simulink model "w3_warplab_agc"  (Simulink 7.7)
settings: Solver=ode45  StartTime=0.0  StopTime=1e4  RelTol=1e-3
PostLoadFcn:
  | w3_warplab_agc_init
InitFcn:
  | w3_warplab_agc_init
StartFcn:
  | w3_warplab_agc_init
values from neighbouring files (symbols this model uses):
  PHY_CONFIG_PKT_DET_CORR_THRESH = 90    [w3_warplab_agc_init.m]
  PHY_CONFIG_PKT_DET_ENERGY_THRESH = 14    [w3_warplab_agc_init.m]
  PHY_CONFIG_PKT_DET_MIN_DURR = 4    [w3_warplab_agc_init.m]
undefined symbols (not defined in the file or in its folder): gcbh, xlBlockLoadCallback, xlGetNormalizedPeriod
libraries: xbsIndex_r4 x1039, xbsEDKLib_r4 x1, simulink x1
(part 3 of 7)

== system w3_warplab_agc/Gain Calc A ==
  I : Inport
  Q : Inport  Port=2
  IQ Valid : Inport  Port=3
  RSSI : Inport  Port=4
  BB gain : Subsystem
  Capture & Convert : Subsystem
  IQ Mag : Subsystem
  RF Gain : Subsystem
  RSSI Avg : Subsystem
  Register{1..4} (4 alike) : xbsIndex_r4/Register  init=0  rst=off  en=off  dbl_ovrd=off  block_type=register
  G_RF : Outport
  G_BB : Outport  Port=2
  wires:
  RF Gain/1(G_RF) -> Register1/1, Capture & Convert/1(G_RF)
  Register1/1 -> Register2/1
  RSSI/1 -> RSSI Avg/1(RSSI)
  RSSI Avg/1(avg) -> Capture & Convert/2(RSSI)
  Capture & Convert/1(Rx Pwr (dBm)) -> RF Gain/1(Rx Pwr), BB gain/2(P_IN_RSSI)
  Register3/1 -> Register4/1
  BB gain/1(G_BB) -> Register3/1
  RF Gain/2(G_RF_dB) -> BB gain/1(G_RF_dB)
  IQ Mag/1(IQ_dBv) -> BB gain/3(IQ_dBv)
  I/1 -> IQ Mag/1(I)
  Q/1 -> IQ Mag/2(Q)
  IQ Valid/1 -> IQ Mag/3(Valid)
  Register2/1 -> G_RF/1
  Register4/1 -> G_BB/1

== system w3_warplab_agc/Gain Calc B ==
  I : Inport
  Q : Inport  Port=2
  IQ Valid : Inport  Port=3
  RSSI : Inport  Port=4
  BB gain : Subsystem
  Capture & Convert : Subsystem
  IQ Mag : Subsystem
  RF Gain : Subsystem
  RSSI Avg : Subsystem
  Register{1..4} (4 alike) : xbsIndex_r4/Register  init=0  rst=off  en=off  dbl_ovrd=off  block_type=register
  G_RF : Outport
  G_BB : Outport  Port=2
  wires:
  Register4/1 -> G_BB/1
  Register2/1 -> G_RF/1
  IQ Valid/1 -> IQ Mag/3(Valid)
  Q/1 -> IQ Mag/2(Q)
  I/1 -> IQ Mag/1(I)
  IQ Mag/1(IQ_dBv) -> BB gain/3(IQ_dBv)
  RF Gain/2(G_RF_dB) -> BB gain/1(G_RF_dB)
  BB gain/1(G_BB) -> Register3/1
  Register3/1 -> Register4/1
  Capture & Convert/1(Rx Pwr (dBm)) -> BB gain/2(P_IN_RSSI), RF Gain/1(Rx Pwr)
  RSSI Avg/1(avg) -> Capture & Convert/2(RSSI)
  RSSI/1 -> RSSI Avg/1(RSSI)
  Register1/1 -> Register2/1
  RF Gain/1(G_RF) -> Capture & Convert/1(G_RF), Register1/1

== system w3_warplab_agc/Gain Calc C ==
  I : Inport
  Q : Inport  Port=2
  IQ Valid : Inport  Port=3
  RSSI : Inport  Port=4
  BB gain : Subsystem
  Capture & Convert : Subsystem
  IQ Mag : Subsystem
  RF Gain : Subsystem
  RSSI Avg : Subsystem
  Register{1..4} (4 alike) : xbsIndex_r4/Register  init=0  rst=off  en=off  dbl_ovrd=off  block_type=register
  G_RF : Outport
  G_BB : Outport  Port=2
  wires:
  RF Gain/1(G_RF) -> Register1/1, Capture & Convert/1(G_RF)
  Register1/1 -> Register2/1
  RSSI/1 -> RSSI Avg/1(RSSI)
  RSSI Avg/1(avg) -> Capture & Convert/2(RSSI)
  Capture & Convert/1(Rx Pwr (dBm)) -> RF Gain/1(Rx Pwr), BB gain/2(P_IN_RSSI)
  Register3/1 -> Register4/1
  BB gain/1(G_BB) -> Register3/1
  RF Gain/2(G_RF_dB) -> BB gain/1(G_RF_dB)
  IQ Mag/1(IQ_dBv) -> BB gain/3(IQ_dBv)
  I/1 -> IQ Mag/1(I)
  Q/1 -> IQ Mag/2(Q)
  IQ Valid/1 -> IQ Mag/3(Valid)
  Register2/1 -> G_RF/1
  Register4/1 -> G_BB/1

== system w3_warplab_agc/Gain Calc D ==
  I : Inport
  Q : Inport  Port=2
  IQ Valid : Inport  Port=3
  RSSI : Inport  Port=4
  BB gain : Subsystem
  Capture & Convert : Subsystem
  IQ Mag : Subsystem
  RF Gain : Subsystem
  RSSI Avg : Subsystem
  Register{1..4} (4 alike) : xbsIndex_r4/Register  init=0  rst=off  en=off  dbl_ovrd=off  block_type=register
  G_RF : Outport
  G_BB : Outport  Port=2
  wires:
  Register4/1 -> G_BB/1
  Register2/1 -> G_RF/1
  IQ Valid/1 -> IQ Mag/3(Valid)
  Q/1 -> IQ Mag/2(Q)
  I/1 -> IQ Mag/1(I)
  IQ Mag/1(IQ_dBv) -> BB gain/3(IQ_dBv)
  RF Gain/2(G_RF_dB) -> BB gain/1(G_RF_dB)
  BB gain/1(G_BB) -> Register3/1
  Register3/1 -> Register4/1
  Capture & Convert/1(Rx Pwr (dBm)) -> BB gain/2(P_IN_RSSI), RF Gain/1(Rx Pwr)
  RSSI Avg/1(avg) -> Capture & Convert/2(RSSI)
  RSSI/1 -> RSSI Avg/1(RSSI)
  Register1/1 -> Register2/1
  RF Gain/1(G_RF) -> Capture & Convert/1(G_RF), Register1/1

== system w3_warplab_agc/IQ Outputs ==
  IQ Valid : Inport
  A I : Inport  Port=2
  A Q : Inport  Port=3
  B I : Inport  Port=4
  B Q : Inport  Port=5
  C I : Inport  Port=6
  C Q : Inport  Port=7
  D I : Inport  Port=8
  D Q : Inport  Port=9
  IQ_Valid_Out : xbsIndex_r4/Gateway Out  inherit_from_input=off  hdl_port=on  timing_constraint=None  locs_specified=off  LOCs={}  UseAsDAC=off  DACChannel='1'  block_type=gatewayout
  RFA_RX_I_OUT : xbsIndex_r4/Gateway Out  inherit_from_input=off  hdl_port=on  timing_constraint=None  locs_specified=off  LOCs={}  UseAsDAC=off  DACChannel='1'  block_type=gatewayout
  RFA_RX_Q_OUT : xbsIndex_r4/Gateway Out  inherit_from_input=off  hdl_port=on  timing_constraint=None  locs_specified=off  LOCs={}  UseAsDAC=off  DACChannel='1'  block_type=gatewayout
  RFB_RX_I_OUT : xbsIndex_r4/Gateway Out  inherit_from_input=off  hdl_port=on  timing_constraint=None  locs_specified=off  LOCs={}  UseAsDAC=off  DACChannel='1'  block_type=gatewayout
  RFB_RX_Q_OUT : xbsIndex_r4/Gateway Out  inherit_from_input=off  hdl_port=on  timing_constraint=None  locs_specified=off  LOCs={}  UseAsDAC=off  DACChannel='1'  block_type=gatewayout
  RFC_RX_I_OUT : xbsIndex_r4/Gateway Out  inherit_from_input=off  hdl_port=on  timing_constraint=None  locs_specified=off  LOCs={}  UseAsDAC=off  DACChannel='1'  block_type=gatewayout
  RFC_RX_Q_OUT : xbsIndex_r4/Gateway Out  inherit_from_input=off  hdl_port=on  timing_constraint=None  locs_specified=off  LOCs={}  UseAsDAC=off  DACChannel='1'  block_type=gatewayout
  RFD_RX_I_OUT : xbsIndex_r4/Gateway Out  inherit_from_input=off  hdl_port=on  timing_constraint=None  locs_specified=off  LOCs={}  UseAsDAC=off  DACChannel='1'  block_type=gatewayout
  RFD_RX_Q_OUT : xbsIndex_r4/Gateway Out  inherit_from_input=off  hdl_port=on  timing_constraint=None  locs_specified=off  LOCs={}  UseAsDAC=off  DACChannel='1'  block_type=gatewayout
  wires:
  A I/1 -> RFA_RX_I_OUT/1
  A Q/1 -> RFA_RX_Q_OUT/1
  IQ Valid/1 -> IQ_Valid_Out/1
  B I/1 -> RFB_RX_I_OUT/1
  B Q/1 -> RFB_RX_Q_OUT/1
  C I/1 -> RFC_RX_I_OUT/1
  C Q/1 -> RFC_RX_Q_OUT/1
  D I/1 -> RFD_RX_I_OUT/1
  D Q/1 -> RFD_RX_Q_OUT/1

== system w3_warplab_agc/RSSI Src ==
  Add : Sum
  Band-Limited White Noise : simulink/Sources/Band-Limited White Noise  SystemSampleTime=-1  Cov=200  Ts=1  seed=abs(ceil(1000*randn))
  Constant : Constant  Value=750
  Down Sample{,1..3} (4 alike) : xbsIndex_r4/Down Sample  sample_ratio=16  sample_phase="Last Value of Frame  (most efficient)"  en=off  latency=1  dbl_ovrd=off  block_type=dsamp
  RFA_RSSI : xbsIndex_r4/Gateway In  gui_display_data_type=Fixed-point  arith_type=Unsigned  n_bits=10  bin_pt=0  preci_type=Single  exp_width=8  frac_width=24  quantization="Round  (unbiased: +/- Inf)"  overflow=Saturate  period=1  dbl_ovrd=off  timing_constraint=None  locs_specified=off  LOCs={}  UseAsADC=off  ADCChannel='1'  inherit_from_input=off  hdl_port=on  block_type=gatewayin
  RFB_RSSI : xbsIndex_r4/Gateway In  gui_display_data_type=Fixed-point  arith_type=Unsigned  n_bits=10  bin_pt=0  preci_type=Single  exp_width=8  frac_width=24  quantization="Round  (unbiased: +/- Inf)"  overflow=Saturate  period=1  dbl_ovrd=off  timing_constraint=None  locs_specified=off  LOCs={}  UseAsADC=off  ADCChannel='1'  inherit_from_input=off  hdl_port=on  block_type=gatewayin
  RFC_RSSI : xbsIndex_r4/Gateway In  gui_display_data_type=Fixed-point  arith_type=Unsigned  n_bits=10  bin_pt=0  preci_type=Single  exp_width=8  frac_width=24  quantization="Round  (unbiased: +/- Inf)"  overflow=Saturate  period=1  dbl_ovrd=off  timing_constraint=None  locs_specified=off  LOCs={}  UseAsADC=off  ADCChannel='1'  inherit_from_input=off  hdl_port=on  block_type=gatewayin
  RFD_RSSI : xbsIndex_r4/Gateway In  gui_display_data_type=Fixed-point  arith_type=Unsigned  n_bits=10  bin_pt=0  preci_type=Single  exp_width=8  frac_width=24  quantization="Round  (unbiased: +/- Inf)"  overflow=Saturate  period=1  dbl_ovrd=off  timing_constraint=None  locs_specified=off  LOCs={}  UseAsADC=off  ADCChannel='1'  inherit_from_input=off  hdl_port=on  block_type=gatewayin
  Register{,1..3} (4 alike) : xbsIndex_r4/Register  init=0  rst=off  en=off  dbl_ovrd=off  block_type=register
  " RFA_RSSI" : Outport
  " RFB_RSSI" : Outport  Port=2
  " RFC_RSSI" : Outport  Port=3
  " RFD_RSSI" : Outport  Port=4
  wires:
  RFA_RSSI/1 -> Register/1
  Register/1 -> Down Sample/1
  Down Sample/1 -> " RFA_RSSI"/1
  Add/1 -> RFA_RSSI/1, RFB_RSSI/1, RFC_RSSI/1, RFD_RSSI/1
  Constant/1 -> Add/1
  Band-Limited White Noise/1 -> Add/2
  RFB_RSSI/1 -> Register1/1
  Register1/1 -> Down Sample1/1
  Down Sample1/1 -> " RFB_RSSI"/1
  RFC_RSSI/1 -> Register2/1
  RFD_RSSI/1 -> Register3/1
  Register2/1 -> Down Sample2/1
  Register3/1 -> Down Sample3/1
  Down Sample3/1 -> " RFD_RSSI"/1
  Down Sample2/1 -> " RFC_RSSI"/1

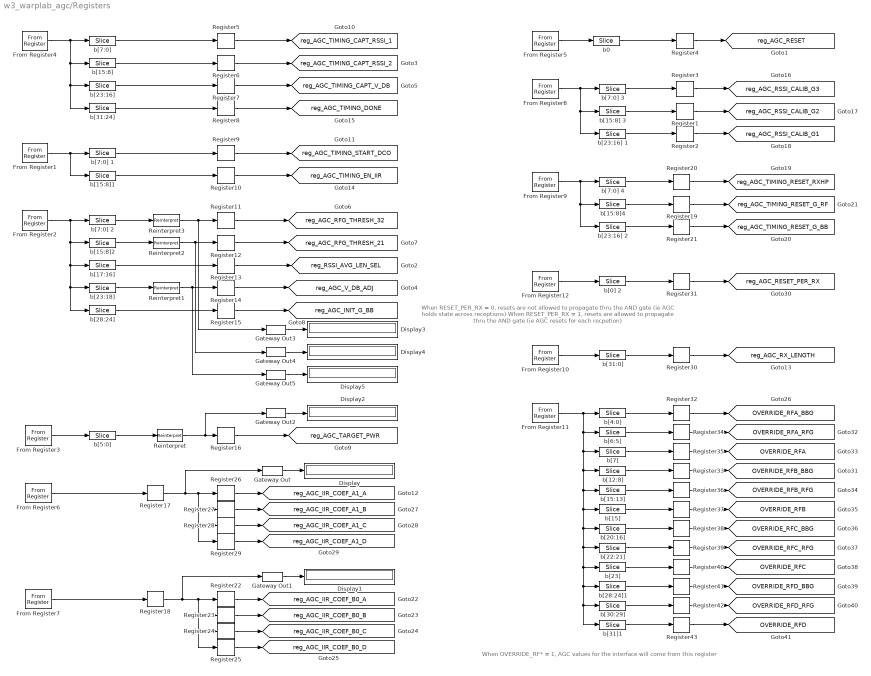
== system w3_warplab_agc/Registers ==
  note: When RESET_PER_RX = 0, resets are not allowed to propagate thru the AND gate (ie AGC holds state across receptions)
      | When RESET_PER_RX = 1, resets are allowed to propagate thru the AND gate (ie AGC resets for each recpetion)
  note: When OVERRIDE_RF* = 1, AGC values for the interface will come from this register
  Display{,1..5} (6 alike) : Display
  From Register1 : xbsIndex_r4/From Register  shared_memory_name='TIMING_DCO'  init=REG_AGC_Timing_DCO  period=1  ownership=Locally owned and initialized  gui_display_data_type=Fixed-point  arith_type=Unsigned  n_bits=32  bin_pt=0  preci_type=Single  dbl_ovrd=off  block_type=fromreg
      settings: AttributesFormatString=<< %<shared_memory_name> >>  infoedit="Register block that reads data to a shared memory register.  Delay of one sample period."
  From Register10 : xbsIndex_r4/From Register  shared_memory_name='RX_LENGTH'  init=REG_AGC_RX_LENGTH  period=1  ownership=Locally owned and initialized  gui_display_data_type=Fixed-point  arith_type=Unsigned  n_bits=32  bin_pt=0  preci_type=Single  dbl_ovrd=off  block_type=fromreg
      settings: AttributesFormatString=<< %<shared_memory_name> >>  infoedit="Register block that reads data to a shared memory register.  Delay of one sample period."
  From Register11 : xbsIndex_r4/From Register  shared_memory_name='AGC_OVERRIDE'  init=REG_ACG_OVERRIDE  period=1  ownership=Locally owned and initialized  gui_display_data_type=Fixed-point  arith_type=Unsigned  n_bits=32  bin_pt=0  preci_type=Single  dbl_ovrd=off  block_type=fromreg
      settings: AttributesFormatString=<< %<shared_memory_name> >>  infoedit="Register block that reads data to a shared memory register.  Delay of one sample period."
  From Register12 : xbsIndex_r4/From Register  shared_memory_name='RESET_MODE'  init=REG_AGC_RESET_MODE  period=1  ownership=Locally owned and initialized  gui_display_data_type=Fixed-point  arith_type=Unsigned  n_bits=32  bin_pt=0  preci_type=Single  dbl_ovrd=off  block_type=fromreg
      settings: AttributesFormatString=<< %<shared_memory_name> >>  infoedit="Register block that reads data to a shared memory register.  Delay of one sample period."
  From Register2 : xbsIndex_r4/From Register  shared_memory_name='CONFIG'  init=REG_AGC_Config  period=1  ownership=Locally owned and initialized  gui_display_data_type=Fixed-point  arith_type=Unsigned  n_bits=32  bin_pt=0  preci_type=Single  dbl_ovrd=off  block_type=fromreg
      settings: AttributesFormatString=<< %<shared_memory_name> >>  infoedit="Register block that reads data to a shared memory register.  Delay of one sample period."
  From Register3 : xbsIndex_r4/From Register  shared_memory_name='TARGET'  init=REG_AGC_Target  period=1  ownership=Locally owned and initialized  gui_display_data_type=Fixed-point  arith_type=Unsigned  n_bits=32  bin_pt=0  preci_type=Single  dbl_ovrd=off  block_type=fromreg
      settings: AttributesFormatString=<< %<shared_memory_name> >>  infoedit="Register block that reads data to a shared memory register.  Delay of one sample period."
  From Register4 : xbsIndex_r4/From Register  shared_memory_name='TIMING_AGC'  init=REG_AGC_Timing_AGC  period=1  ownership=Locally owned and initialized  gui_display_data_type=Fixed-point  arith_type=Unsigned  n_bits=32  bin_pt=0  preci_type=Single  dbl_ovrd=off  block_type=fromreg
      settings: AttributesFormatString=<< %<shared_memory_name> >>  infoedit="Register block that reads data to a shared memory register.  Delay of one sample period."
  From Register5 : xbsIndex_r4/From Register  shared_memory_name='RESET'  init=0  period=1  ownership=Locally owned and initialized  gui_display_data_type=Fixed-point  arith_type=Unsigned  n_bits=32  bin_pt=0  preci_type=Single  dbl_ovrd=off  block_type=fromreg
      settings: AttributesFormatString=<< %<shared_memory_name> >>  infoedit="Register block that reads data to a shared memory register.  Delay of one sample period."
  From Register6 : xbsIndex_r4/From Register  shared_memory_name='IIR_COEF_A1'  init=REG_AGC_IIR_Coef_A1  period=1  ownership=Locally owned and initialized  gui_display_data_type=Fixed-point  arith_type="Signed  (2's comp)"  n_bits=18  bin_pt=17  preci_type=Single  dbl_ovrd=off  block_type=fromreg
      settings: AttributesFormatString=<< %<shared_memory_name> >>  infoedit="Register block that reads data to a shared memory register.  Delay of one sample period."
  From Register7 : xbsIndex_r4/From Register  shared_memory_name='IIR_COEF_B0'  init=REG_AGC_IIR_Coef_B0  period=1  ownership=Locally owned and initialized  gui_display_data_type=Fixed-point  arith_type=Unsigned  n_bits=18  bin_pt=17  preci_type=Single  dbl_ovrd=off  block_type=fromreg
      settings: AttributesFormatString=<< %<shared_memory_name> >>  infoedit="Register block that reads data to a shared memory register.  Delay of one sample period."
  From Register8 : xbsIndex_r4/From Register  shared_memory_name='RSSI_PWR_CALIB'  init=REG_AGC_RSSI_RX_PWR_CALIB  period=1  ownership=Locally owned and initialized  gui_display_data_type=Fixed-point  arith_type=Unsigned  n_bits=32  bin_pt=0  preci_type=Single  dbl_ovrd=off  block_type=fromreg
      settings: AttributesFormatString=<< %<shared_memory_name> >>  infoedit="Register block that reads data to a shared memory register.  Delay of one sample period."
  From Register9 : xbsIndex_r4/From Register  shared_memory_name='TIMING_RESET'  init=REG_AGC_Timing_Reset  period=1  ownership=Locally owned and initialized  gui_display_data_type=Fixed-point  arith_type=Unsigned  n_bits=32  bin_pt=0  preci_type=Single  dbl_ovrd=off  block_type=fromreg
      settings: AttributesFormatString=<< %<shared_memory_name> >>  infoedit="Register block that reads data to a shared memory register.  Delay of one sample period."
  Gateway Out{,1..5} (6 alike) : xbsIndex_r4/Gateway Out  inherit_from_input=off  hdl_port=off  timing_constraint=None  locs_specified=off  LOCs={}  UseAsDAC=off  DACChannel='1'  block_type=gatewayout
  Register{1..43} (43 alike) : xbsIndex_r4/Register  init=0  rst=off  en=off  dbl_ovrd=off  block_type=register
  Reinterpret{,1..3} (4 alike) : xbsIndex_r4/Reinterpret  force_arith_type=on  arith_type="Signed  (2's comp)"  force_bin_pt=off  bin_pt=0  block_type=reinterpret
  b0 : xbsIndex_r4/Slice  nbits=1  boolean_output=on  mode=Lower Bit Location + Width  bit1=0  base1=MSB of Input  bit0=0  base0=LSB of Input  dbl_ovrd=off  block_type=slice
      settings: block_version=VER_STRING_GOES_HERE
  b[0] 2 : xbsIndex_r4/Slice  nbits=1  boolean_output=off  mode=Lower Bit Location + Width  bit1=0  base1=MSB of Input  bit0=0  base0=LSB of Input  dbl_ovrd=off  block_type=slice
      settings: block_version=VER_STRING_GOES_HERE
  b[12:8] : xbsIndex_r4/Slice  nbits=5  boolean_output=off  mode=Lower Bit Location + Width  bit1=0  base1=MSB of Input  bit0=8  base0=LSB of Input  dbl_ovrd=off  block_type=slice
      settings: block_version=VER_STRING_GOES_HERE
  b[15:13] : xbsIndex_r4/Slice  nbits=2  boolean_output=off  mode=Lower Bit Location + Width  bit1=0  base1=MSB of Input  bit0=13  base0=LSB of Input  dbl_ovrd=off  block_type=slice
      settings: block_version=VER_STRING_GOES_HERE
  b[15:8]{,1..2,4} (4 alike) : xbsIndex_r4/Slice  nbits=8  boolean_output=off  mode=Lower Bit Location + Width  bit1=0  base1=MSB of Input  bit0=8  base0=LSB of Input  dbl_ovrd=off  block_type=slice
      settings: block_version=VER_STRING_GOES_HERE
  b[15:8] 3 : xbsIndex_r4/Slice  nbits=8  boolean_output=off  mode=Lower Bit Location + Width  bit1=0  base1=MSB of Input  bit0=8  base0=LSB of Input  dbl_ovrd=off  block_type=slice
      settings: block_version=VER_STRING_GOES_HERE
  b[15] : xbsIndex_r4/Slice  nbits=1  boolean_output=off  mode=Lower Bit Location + Width  bit1=0  base1=MSB of Input  bit0=15  base0=LSB of Input  dbl_ovrd=off  block_type=slice
      settings: block_version=VER_STRING_GOES_HERE
  b[17:16] : xbsIndex_r4/Slice  nbits=2  boolean_output=off  mode=Lower Bit Location + Width  bit1=0  base1=MSB of Input  bit0=16  base0=LSB of Input  dbl_ovrd=off  block_type=slice
      settings: block_version=VER_STRING_GOES_HERE
  b[20:16] : xbsIndex_r4/Slice  nbits=5  boolean_output=off  mode=Lower Bit Location + Width  bit1=0  base1=MSB of Input  bit0=16  base0=LSB of Input  dbl_ovrd=off  block_type=slice
      settings: block_version=VER_STRING_GOES_HERE
  b[22:21] : xbsIndex_r4/Slice  nbits=2  boolean_output=off  mode=Lower Bit Location + Width  bit1=0  base1=MSB of Input  bit0=21  base0=LSB of Input  dbl_ovrd=off  block_type=slice
      settings: block_version=VER_STRING_GOES_HERE
  b[23:16] : xbsIndex_r4/Slice  nbits=8  boolean_output=off  mode=Lower Bit Location + Width  bit1=0  base1=MSB of Input  bit0=16  base0=LSB of Input  dbl_ovrd=off  block_type=slice
      settings: block_version=VER_STRING_GOES_HERE
  b[23:16] 1 : xbsIndex_r4/Slice  nbits=8  boolean_output=off  mode=Lower Bit Location + Width  bit1=0  base1=MSB of Input  bit0=16  base0=LSB of Input  dbl_ovrd=off  block_type=slice
      settings: block_version=VER_STRING_GOES_HERE
  b[23:16] 2 : xbsIndex_r4/Slice  nbits=8  boolean_output=off  mode=Lower Bit Location + Width  bit1=0  base1=MSB of Input  bit0=16  base0=LSB of Input  dbl_ovrd=off  block_type=slice
      settings: block_version=VER_STRING_GOES_HERE
  b[23:18] : xbsIndex_r4/Slice  nbits=6  boolean_output=off  mode=Lower Bit Location + Width  bit1=0  base1=MSB of Input  bit0=18  base0=LSB of Input  dbl_ovrd=off  block_type=slice
      settings: block_version=VER_STRING_GOES_HERE
  b[23] : xbsIndex_r4/Slice  nbits=1  boolean_output=off  mode=Lower Bit Location + Width  bit1=0  base1=MSB of Input  bit0=23  base0=LSB of Input  dbl_ovrd=off  block_type=slice
      settings: block_version=VER_STRING_GOES_HERE
  b[28:24] : xbsIndex_r4/Slice  nbits=5  boolean_output=off  mode=Lower Bit Location + Width  bit1=0  base1=MSB of Input  bit0=24  base0=LSB of Input  dbl_ovrd=off  block_type=slice
      settings: block_version=VER_STRING_GOES_HERE
  b[28:24]1 : xbsIndex_r4/Slice  nbits=5  boolean_output=off  mode=Lower Bit Location + Width  bit1=0  base1=MSB of Input  bit0=24  base0=LSB of Input  dbl_ovrd=off  block_type=slice
      settings: block_version=VER_STRING_GOES_HERE
  b[30:29] : xbsIndex_r4/Slice  nbits=2  boolean_output=off  mode=Lower Bit Location + Width  bit1=0  base1=MSB of Input  bit0=29  base0=LSB of Input  dbl_ovrd=off  block_type=slice
      settings: block_version=VER_STRING_GOES_HERE
  b[31:0] : xbsIndex_r4/Slice  nbits=32  boolean_output=off  mode=Lower Bit Location + Width  bit1=0  base1=MSB of Input  bit0=0  base0=LSB of Input  dbl_ovrd=off  block_type=slice
      settings: block_version=VER_STRING_GOES_HERE
  b[31:24] : xbsIndex_r4/Slice  nbits=8  boolean_output=off  mode=Lower Bit Location + Width  bit1=0  base1=MSB of Input  bit0=24  base0=LSB of Input  dbl_ovrd=off  block_type=slice
      settings: block_version=VER_STRING_GOES_HERE
  b[31]1 : xbsIndex_r4/Slice  nbits=1  boolean_output=off  mode=Lower Bit Location + Width  bit1=0  base1=MSB of Input  bit0=31  base0=LSB of Input  dbl_ovrd=off  block_type=slice
      settings: block_version=VER_STRING_GOES_HERE
  b[4:0] : xbsIndex_r4/Slice  nbits=5  boolean_output=off  mode=Lower Bit Location + Width  bit1=0  base1=MSB of Input  bit0=0  base0=LSB of Input  dbl_ovrd=off  block_type=slice
      settings: block_version=VER_STRING_GOES_HERE
  b[5:0] : xbsIndex_r4/Slice  nbits=6  boolean_output=off  mode=Lower Bit Location + Width  bit1=0  base1=MSB of Input  bit0=0  base0=LSB of Input  dbl_ovrd=off  block_type=slice
      settings: block_version=VER_STRING_GOES_HERE
  b[6:5] : xbsIndex_r4/Slice  nbits=2  boolean_output=off  mode=Lower Bit Location + Width  bit1=0  base1=MSB of Input  bit0=5  base0=LSB of Input  dbl_ovrd=off  block_type=slice
      settings: block_version=VER_STRING_GOES_HERE
  b[7:0] {,1..4} (5 alike) : xbsIndex_r4/Slice  nbits=8  boolean_output=off  mode=Lower Bit Location + Width  bit1=0  base1=MSB of Input  bit0=0  base0=LSB of Input  dbl_ovrd=off  block_type=slice
      settings: block_version=VER_STRING_GOES_HERE
  b[7] : xbsIndex_r4/Slice  nbits=1  boolean_output=off  mode=Lower Bit Location + Width  bit1=0  base1=MSB of Input  bit0=7  base0=LSB of Input  dbl_ovrd=off  block_type=slice
      settings: block_version=VER_STRING_GOES_HERE
  tag scope: OVERRIDE_RFA=global, OVERRIDE_RFA_BBG=global, OVERRIDE_RFA_RFG=global, OVERRIDE_RFB=global, OVERRIDE_RFB_BBG=global, OVERRIDE_RFB_RFG=global, OVERRIDE_RFC=global, OVERRIDE_RFC_BBG=global, OVERRIDE_RFC_RFG=global, OVERRIDE_RFD=global, OVERRIDE_RFD_BBG=global, OVERRIDE_RFD_RFG=global, reg_AGC_IIR_COEF_A1_A=global, reg_AGC_IIR_COEF_A1_B=global, reg_AGC_IIR_COEF_A1_C=global, reg_AGC_IIR_COEF_A1_D=global, reg_AGC_IIR_COEF_B0_A=global, reg_AGC_IIR_COEF_B0_B=global, reg_AGC_IIR_COEF_B0_C=global, reg_AGC_IIR_COEF_B0_D=global, reg_AGC_INIT_G_BB=global, reg_AGC_RESET=global, reg_AGC_RESET_PER_RX=global, reg_AGC_RFG_THRESH_21=global, reg_AGC_RFG_THRESH_32=global, reg_AGC_RSSI_CALIB_G1=global, reg_AGC_RSSI_CALIB_G2=global, reg_AGC_RSSI_CALIB_G3=global, reg_AGC_RX_LENGTH=global, reg_AGC_TARGET_PWR=global, reg_AGC_TIMING_CAPT_RSSI_1=global, reg_AGC_TIMING_CAPT_RSSI_2=global, reg_AGC_TIMING_CAPT_V_DB=global, reg_AGC_TIMING_DONE=global, reg_AGC_TIMING_EN_IIR=global, reg_AGC_TIMING_RESET_G_BB=global, reg_AGC_TIMING_RESET_G_RF=global, reg_AGC_TIMING_RESET_RXHP=global, reg_AGC_TIMING_START_DCO=global, reg_AGC_V_DB_ADJ=global, reg_RSSI_AVG_LEN_SEL=global
  wires:
  From Register4/1 -> "b[7:0] "/1, b[15:8]/1, b[23:16]/1, b[31:24]/1
  "b[7:0] "/1 -> Register5/1
  b[15:8]/1 -> Register6/1
  b[23:16]/1 -> Register7/1
  From Register1/1 -> b[7:0] 1/1, b[15:8]1/1
  b[7:0] 1/1 -> Register9/1
  b[15:8]1/1 -> Register10/1
  From Register2/1 -> b[15:8]2/1, b[17:16]/1, b[23:18]/1, b[28:24]/1, b[7:0] 2/1
  b[7:0] 2/1 -> Reinterpret3/1
  b[15:8]2/1 -> Reinterpret2/1
  b[17:16]/1 -> Register13/1
  b[23:18]/1 -> Reinterpret1/1
  b[28:24]/1 -> Register15/1
  From Register3/1 -> b[5:0]/1
  b[5:0]/1 -> Reinterpret/1
  Reinterpret/1 -> Gateway Out2/1, Register16/1
  Reinterpret1/1 -> Gateway Out5/1, Register14/1
  Reinterpret2/1 -> Gateway Out4/1, Register12/1
  Reinterpret3/1 -> Gateway Out3/1, Register11/1
  From Register5/1 -> b0/1
  b0/1 -> Register4/1
  From Register6/1 -> Register17/1
  From Register7/1 -> Register18/1
  Gateway Out/1 -> Display/1
  Gateway Out1/1 -> Display1/1
  Gateway Out2/1 -> Display2/1
  Gateway Out3/1 -> Display3/1
  Gateway Out4/1 -> Display4/1
  Gateway Out5/1 -> Display5/1
  b[31:24]/1 -> Register8/1
  From Register8/1 -> b[15:8] 3/1, b[23:16] 1/1, b[7:0] 3/1
  b[7:0] 3/1 -> Register3/1
  b[15:8] 3/1 -> Register1/1
  b[23:16] 1/1 -> Register2/1
  Register3/1 -> [reg_AGC_RSSI_CALIB_G3]
  Register1/1 -> [reg_AGC_RSSI_CALIB_G2]
  Register2/1 -> [reg_AGC_RSSI_CALIB_G1]
  Register4/1 -> [reg_AGC_RESET]
  Register5/1 -> [reg_AGC_TIMING_CAPT_RSSI_1]
  Register6/1 -> [reg_AGC_TIMING_CAPT_RSSI_2]
  Register7/1 -> [reg_AGC_TIMING_CAPT_V_DB]
  Register8/1 -> [reg_AGC_TIMING_DONE]
  Register9/1 -> [reg_AGC_TIMING_START_DCO]
  Register10/1 -> [reg_AGC_TIMING_EN_IIR]
  Register11/1 -> [reg_AGC_RFG_THRESH_32]
  Register12/1 -> [reg_AGC_RFG_THRESH_21]
  Register13/1 -> [reg_RSSI_AVG_LEN_SEL]
  Register14/1 -> [reg_AGC_V_DB_ADJ]
  Register15/1 -> [reg_AGC_INIT_G_BB]
  Register16/1 -> [reg_AGC_TARGET_PWR]
  Register17/1 -> Gateway Out/1, Register28/1, Register29/1, Register27/1, Register26/1
  Register18/1 -> Gateway Out1/1, Register24/1, Register25/1, Register23/1, Register22/1
  From Register9/1 -> b[7:0] 4/1, b[15:8]4/1, b[23:16] 2/1
  b[7:0] 4/1 -> Register20/1
  b[15:8]4/1 -> Register19/1
  Register20/1 -> [reg_AGC_TIMING_RESET_RXHP]
  Register19/1 -> [reg_AGC_TIMING_RESET_G_RF]
  b[23:16] 2/1 -> Register21/1
  Register21/1 -> [reg_AGC_TIMING_RESET_G_BB]
  Register22/1 -> [reg_AGC_IIR_COEF_B0_A]
  Register23/1 -> [reg_AGC_IIR_COEF_B0_B]
  Register24/1 -> [reg_AGC_IIR_COEF_B0_C]
  Register25/1 -> [reg_AGC_IIR_COEF_B0_D]
  Register26/1 -> [reg_AGC_IIR_COEF_A1_A]
  Register27/1 -> [reg_AGC_IIR_COEF_A1_B]
  Register28/1 -> [reg_AGC_IIR_COEF_A1_C]
  Register29/1 -> [reg_AGC_IIR_COEF_A1_D]
  From Register10/1 -> b[31:0]/1
  b[31:0]/1 -> Register30/1
  b[0] 2/1 -> Register31/1
  Register30/1 -> [reg_AGC_RX_LENGTH]
  Register31/1 -> [reg_AGC_RESET_PER_RX]
  From Register11/1 -> b[4:0]/1, b[6:5]/1, b[7]/1, b[12:8]/1, b[15:13]/1, b[15]/1, b[20:16]/1, b[22:21]/1, b[23]/1, b[28:24]1/1, b[30:29]/1, b[31]1/1
  b[4:0]/1 -> Register32/1
  Register32/1 -> [OVERRIDE_RFA_BBG]
  b[6:5]/1 -> Register34/1
  Register34/1 -> [OVERRIDE_RFA_RFG]
  b[7]/1 -> Register35/1
  Register35/1 -> [OVERRIDE_RFA]
  b[12:8]/1 -> Register33/1
  Register33/1 -> [OVERRIDE_RFB_BBG]
  b[15:13]/1 -> Register36/1
  Register36/1 -> [OVERRIDE_RFB_RFG]
  b[15]/1 -> Register37/1
  Register37/1 -> [OVERRIDE_RFB]
  b[20:16]/1 -> Register38/1
  Register38/1 -> [OVERRIDE_RFC_BBG]
  b[22:21]/1 -> Register39/1
  Register39/1 -> [OVERRIDE_RFC_RFG]
  b[23]/1 -> Register40/1
  Register40/1 -> [OVERRIDE_RFC]
  b[28:24]1/1 -> Register41/1
  Register41/1 -> [OVERRIDE_RFD_BBG]
  b[30:29]/1 -> Register42/1
  Register42/1 -> [OVERRIDE_RFD_RFG]
  b[31]1/1 -> Register43/1
  Register43/1 -> [OVERRIDE_RFD]
  From Register12/1 -> b[0] 2/1

== system w3_warplab_agc/S-R Latch ==
  S : Inport
  R : Inport  Port=2
  Constant1 : xbsIndex_r4/Constant  const=1  gui_display_data_type=Boolean  arith_type=Boolean  n_bits=1  bin_pt=0  preci_type=Single  exp_width=8  frac_width=24  explicit_period=off  period=1  equ=P=C  opselect=C  inp2=PCIN>>17  opr=+  inp1=P  carry=CIN  dbl_ovrd=off  block_type=constant
      settings: block_version=VER_STRING_GOES_HERE
  Convert1 : xbsIndex_r4/Convert  gui_display_data_type=Boolean  arith_type=Boolean  n_bits=1  bin_pt=0  float_type=Single  exp_bits=8  fraction_bits=24  quantization=Truncate  overflow=Wrap  en=off  latency=0  dbl_ovrd=off  pipeline=off  block_type=convert
  Convert2 : xbsIndex_r4/Convert  gui_display_data_type=Boolean  arith_type=Boolean  n_bits=1  bin_pt=0  float_type=Single  exp_bits=8  fraction_bits=24  quantization=Truncate  overflow=Wrap  en=off  latency=0  dbl_ovrd=off  pipeline=off  block_type=convert
  Register2 : xbsIndex_r4/Register  init=0  rst=on  en=on  dbl_ovrd=off  block_type=register
      settings: xl_area=[1 1 0 0 0 0 0]  block_version=VER_STRING_GOES_HERE
  Q : Outport
  wires:
  Convert2/1 -> Register2/3
  Convert1/1 -> Register2/2
  Constant1/1 -> Register2/1
  R/1 -> Convert1/1
  Register2/1 -> Q/1
  S/1 -> Convert2/1

== system w3_warplab_agc/ADC Inputs/negedge1 ==
  D : Inport
  Delay : xbsIndex_r4/Delay  rst=off  infoeditControl=Selection of Reset will increase slice count due to use of real FFs and instead of SRLs  en=off  latency=1  dbl_ovrd=off  reg_retiming=off  block_type=delay
      settings: infoedit=Hardware notes: A delay line is a chain, each link of which is an SRL16 followed by a flip-flop. If register retiming is enabled, the delay line is a chain of flip-flops.  xl_area=[1 1 0 0 0 0 0]  block_version=VER_STRING_GOES_HERE
  Inverter : xbsIndex_r4/Inverter  en=off  latency=0  dbl_ovrd=off  block_type=inv
      settings: xl_area=[0 0 0 0 0 0 0]  block_version=VER_STRING_GOES_HERE
  Logical1 : xbsIndex_r4/Logical  logical_function=AND  inputs=2  en=off  latency=0  precision=Full  arith_type=Unsigned  n_bits=8  bin_pt=2  align_bp=on  dbl_ovrd=off  block_type=logical
      settings: xl_area=[1 0 0 1 0 0 0]  block_version=VER_STRING_GOES_HERE
  Q : Outport
  wires:
  D/1 -> Delay/1, Inverter/1
  Logical1/1 -> Q/1
  Delay/1 -> Logical1/1
  Inverter/1 -> Logical1/2

== system w3_warplab_agc/Auto-Corr Pkt Det/Auto Corr ==
  Valid : Inport
  I : Inport  Port=2
  Q : Inport  Port=3
  Avg Mag : Subsystem
  Conj Mult : Subsystem
  Delay : xbsIndex_r4/Delay  rst=off  infoeditControl=Selection of Reset will increase slice count due to use of real FFs and instead of SRLs  en=on  latency=16  dbl_ovrd=off  reg_retiming=off  block_type=delay
      settings: xl_area=[7 14 0 14 0 0 0]  block_version=VER_STRING_GOES_HERE
  Delay1 : xbsIndex_r4/Delay  rst=off  infoeditControl=Selection of Reset will increase slice count due to use of real FFs and instead of SRLs  en=on  latency=16  dbl_ovrd=off  reg_retiming=off  block_type=delay
      settings: xl_area=[7 14 0 14 0 0 0]  block_version=VER_STRING_GOES_HERE
  Corr : Outport
  wires:
  I/1 -> Delay/1, Conj Mult/2(A I)
  Q/1 -> Delay1/1, Conj Mult/3(A Q)
  Delay/1 -> Conj Mult/4(B I)
  Delay1/1 -> Conj Mult/5(B Q)
  Valid/1 -> Conj Mult/1(Valid), Delay1/2, Delay/2
  Conj Mult/2(" I") -> Avg Mag/2(I)
  Conj Mult/3(" Q") -> Avg Mag/3(Q)
  Conj Mult/1(" Valid") -> Avg Mag/1(Valid)
  Avg Mag/1(M) -> Corr/1

== system w3_warplab_agc/Auto-Corr Pkt Det/Decision ==
  PktDet Reset : Inport
  Corr : Inport  Port=2
  Mag : Inport  Port=3
  Display{,1..3} (4 alike) : Display
  Logical : xbsIndex_r4/Logical  logical_function=AND  inputs=2  en=off  latency=0  precision=Full  arith_type=Unsigned  n_bits=8  bin_pt=2  align_bp=on  dbl_ovrd=off  block_type=logical
      settings: xl_area=[1 0 0 1 0 0 0]  block_version=VER_STRING_GOES_HERE
  Min Dur : Subsystem
  Mult1 : xbsIndex_r4/Mult  precision=User Defined  arith_type=Unsigned  n_bits=30  bin_pt=20  quantization=Truncate  overflow=Flag as error  en=off  latency=1  dbl_ovrd=off  use_behavioral_HDL=off  opt=Speed  use_embedded=on  optimum_pipeline=off  pipeline=on  use_rpm=off  placement_style=Rectangular shape  block_type=mult
      settings: xl_area=[63 105 0 106 0 4 0]  block_version=VER_STRING_GOES_HERE
  Reinterpret : xbsIndex_r4/Reinterpret  force_arith_type=on  arith_type=Unsigned  force_bin_pt=on  bin_pt=0  block_type=reinterpret
  Reinterpret1 : xbsIndex_r4/Reinterpret  force_arith_type=on  arith_type=Unsigned  force_bin_pt=on  bin_pt=0  block_type=reinterpret
  Relational : xbsIndex_r4/Relational  mode=a>b  en=off  latency=1  dbl_ovrd=off  block_type=relational
      settings: xl_area=[11 1 0 22 0 0 0]  block_version=VER_STRING_GOES_HERE
  Relational1 : xbsIndex_r4/Relational  mode=a>b  en=off  latency=1  dbl_ovrd=off  block_type=relational
      settings: xl_area=[11 1 0 22 0 0 0]  block_version=VER_STRING_GOES_HERE
  done{14..15,17..18} (4 alike) : xbsIndex_r4/Gateway Out  inherit_from_input=off  hdl_port=off  timing_constraint=None  locs_specified=off  LOCs={}  UseAsDAC=off  DACChannel='1'  block_type=gatewayout
      settings: infoedit="Gateway out block.  Converts Xilinx fixed point inputs into ouputs of type Simulink integer, double, or fixed point.<P><P>Hardware notes:  In hardware these blocks become top level output ports or are discarded, depending on how they are configured."  xl_area=[0 0 0 0 1 0 0]  block_version=VER_STRING_GOES_HERE
  PktDet : Outport
  wires:
  done18/1 -> Display3/1
  Reinterpret1/1 -> done18/1
  done17/1 -> Display2/1
  Reinterpret/1 -> done17/1
  done15/1 -> Display1/1
  done14/1 -> Display/1
  [regRx_PktDet_CorrThresh] -> Reinterpret/1, done14/1
  [regRx_PktDet_EnergyThresh] -> Reinterpret1/1, done15/1
  Corr/1 -> Relational/1
  Mag/1 -> Mult1/2, Relational1/1
  [regRx_PktDet_CorrThresh] -> Mult1/1
  Mult1/1 -> Relational/2
  [regRx_PktDet_EnergyThresh] -> Relational1/2
  Logical/1 -> Min Dur/1(Det)
  PktDet Reset/1 -> Min Dur/2(Reset)
  Min Dur/1(Pkt Det) -> PktDet/1
  Relational/1 -> Logical/1
  Relational1/1 -> Logical/2

== system w3_warplab_agc/Auto-Corr Pkt Det/Mag ==
  Valid : Inport
  I : Inport  Port=2
  Q : Inport  Port=3
  AddSub : xbsIndex_r4/AddSub  mode=Addition  use_carryin=off  use_carryout=off  en=off  latency=0  precision=User Defined  arith_type="Signed  (2's comp)"  n_bits=20  bin_pt=18  quantization=Truncate  overflow=Flag as error  dbl_ovrd=off  use_behavioral_HDL=off  hw_selection=Fabric  pipelined=off  block_type=addsub
  Delay : xbsIndex_r4/Delay  rst=off  infoeditControl=Selection of Reset will increase slice count due to use of real FFs and instead of SRLs  en=off  latency=1  dbl_ovrd=off  reg_retiming=off  block_type=delay
  Mult : xbsIndex_r4/Mult  precision=User Defined  arith_type="Signed  (2's comp)"  n_bits=20  bin_pt=19  quantization=Truncate  overflow=Saturate  en=off  latency=1  dbl_ovrd=off  use_behavioral_HDL=off  opt=Speed  use_embedded=on  optimum_pipeline=off  pipeline=on  use_rpm=on  placement_style=Triangular  block_type=mult
  Mult1 : xbsIndex_r4/Mult  precision=User Defined  arith_type="Signed  (2's comp)"  n_bits=20  bin_pt=19  quantization=Truncate  overflow=Saturate  en=off  latency=1  dbl_ovrd=off  use_behavioral_HDL=off  opt=Speed  use_embedded=on  optimum_pipeline=off  pipeline=on  use_rpm=on  placement_style=Triangular  block_type=mult
  Mult2 : xbsIndex_r4/Mult  precision=User Defined  arith_type="Signed  (2's comp)"  n_bits=25  bin_pt=18  quantization=Truncate  overflow=Saturate  en=on  latency=1  dbl_ovrd=off  use_behavioral_HDL=off  opt=Speed  use_embedded=on  optimum_pipeline=off  pipeline=on  use_rpm=on  placement_style=Triangular  block_type=mult
  Running Sum : Subsystem
  Mag Sq : Outport
  Mag : Outport  Port=2
  wires:
  Delay/1 -> Running Sum/1(En)
  I/1 -> Mult/1, Mult/2
  Valid/1 -> Delay/1
  Running Sum/1(Sum) -> Mult2/1, Mult2/2, Mag/1
  Q/1 -> Mult1/1, Mult1/2
  Mult/1 -> AddSub/1
  Mult1/1 -> AddSub/2
  AddSub/1 -> Running Sum/2(D)
  Mult2/1 -> Mag Sq/1
  Running Sum/2(Valid) -> Mult2/3

== system w3_warplab_agc/Ctrl/Done Generator ==
  note: AGC Sample Counter: resets agc after some number of samples (defined by RX_LENGTH register)
  note: NOTE:  The AGC_RESET signal will reset all downstream paths.  Therefore,
      | we do not need to generate a done signal on an AGC_RESET, merely reset
      | the current timeout counter because everything else will be gracefully reset.
  note: NOTE:  Since the reset has precedence over the set, we have to delay
      | by a cycle so that the run will be triggered even when the core is in reset
  IQ Valid : Inport
  Run : Inport  Port=2
  Convert : xbsIndex_r4/Convert  gui_display_data_type=Boolean  arith_type=Boolean  n_bits=16  bin_pt=14  float_type=Single  exp_bits=8  fraction_bits=24  quantization=Truncate  overflow=Wrap  en=off  latency=0  dbl_ovrd=off  pipeline=off  block_type=convert
      settings: block_version=8.2
  Convert1 : xbsIndex_r4/Convert  gui_display_data_type=Boolean  arith_type=Boolean  n_bits=16  bin_pt=14  float_type=Single  exp_bits=8  fraction_bits=24  quantization=Truncate  overflow=Wrap  en=off  latency=0  dbl_ovrd=off  pipeline=off  block_type=convert
      settings: block_version=8.2
  Inverter2 : xbsIndex_r4/Inverter  en=off  latency=0  dbl_ovrd=off  block_type=inv
      settings: xl_area=[0 0 0 0 0 0 0]  block_version=VER_STRING_GOES_HERE
  Logical3 : xbsIndex_r4/Logical  logical_function=AND  inputs=2  en=off  latency=0  precision=Full  arith_type=Unsigned  n_bits=16  bin_pt=0  align_bp=on  dbl_ovrd=off  block_type=logical
  Logical4 : xbsIndex_r4/Logical  logical_function=AND  inputs=3  en=off  latency=0  precision=Full  arith_type=Unsigned  n_bits=16  bin_pt=0  align_bp=on  dbl_ovrd=off  block_type=logical
      settings: xl_area=[1 0 0 1 0 0 0]  block_version=VER_STRING_GOES_HERE
  Register8 : xbsIndex_r4/Register  init=0  rst=off  en=off  dbl_ovrd=off  block_type=register
  Relational4 : xbsIndex_r4/Relational  mode=a>=b  en=off  latency=0  dbl_ovrd=off  block_type=relational
      settings: xl_area=[5 0 0 9 0 0 0]  block_version=VER_STRING_GOES_HERE
  RisingEdge : Subsystem
  S-R Latch1 : Subsystem
  sample_count : xbsIndex_r4/Counter  cnt_type=Free Running  cnt_to=Inf  operation=Up  start_count=0  cnt_by_val=1  arith_type=Unsigned  n_bits=32  bin_pt=0  load_pin=off  rst=on  en=on  explicit_period=on  period=1  dbl_ovrd=off  use_behavioral_HDL=off  implementation=Fabric  use_rpm=off  block_type=counter
      settings: xl_area=[10 18 0 18 0 0 0]  block_version=VER_STRING_GOES_HERE
  Done : Outport
  wires:
  Run/1 -> Register8/1
  [AGC_RESET] -> S-R Latch1/2(R), sample_count/1
  [reg_AGC_RESET_PER_RX] -> Convert1/1
  Logical4/1 -> sample_count/2
  sample_count/1 -> Relational4/1
  Relational4/1 -> Inverter2/1, RisingEdge/1(IN)
  Inverter2/1 -> Logical4/1
  [reg_AGC_RX_LENGTH] -> Relational4/2
  RisingEdge/1(Edge) -> Convert/1
  Convert/1 -> Logical3/1
  Convert1/1 -> Logical3/2
  Logical3/1 -> Done/1
  IQ Valid/1 -> Logical4/2
  S-R Latch1/1(Q) -> Logical4/3
  Register8/1 -> S-R Latch1/1(S)

== system w3_warplab_agc/Ctrl/Posedge0 ==
  note: Rising Edge Detection
  D : Inport
  Delay : xbsIndex_r4/Delay  rst=off  infoeditControl=Selection of Reset will increase slice count due to use of real FFs and instead of SRLs  en=off  latency=1  dbl_ovrd=off  reg_retiming=off  block_type=delay
      settings: infoedit=Hardware notes: A delay line is a chain, each link of which is an SRL16 followed by a flip-flop. If register retiming is enabled, the delay line is a chain of flip-flops.  xl_area=[1 1 0 0 0 0 0]  block_version=VER_STRING_GOES_HERE
  Inverter : xbsIndex_r4/Inverter  en=off  latency=0  dbl_ovrd=off  block_type=inv
      settings: xl_area=[0 0 0 0 0 0 0]  block_version=VER_STRING_GOES_HERE
  Logical1 : xbsIndex_r4/Logical  logical_function=AND  inputs=2  en=off  latency=0  precision=Full  arith_type=Unsigned  n_bits=8  bin_pt=2  align_bp=on  dbl_ovrd=off  block_type=logical
      settings: xl_area=[1 0 0 1 0 0 0]  block_version=VER_STRING_GOES_HERE
  Q : Outport
  wires:
  D/1 -> Logical1/2, Delay/1
  Logical1/1 -> Q/1
  Inverter/1 -> Logical1/1
  Delay/1 -> Inverter/1

== system w3_warplab_agc/Ctrl/Posedge1 ==
  note: Rising Edge Detection
  D : Inport
  Delay : xbsIndex_r4/Delay  rst=off  infoeditControl=Selection of Reset will increase slice count due to use of real FFs and instead of SRLs  en=off  latency=1  dbl_ovrd=off  reg_retiming=off  block_type=delay
      settings: infoedit=Hardware notes: A delay line is a chain, each link of which is an SRL16 followed by a flip-flop. If register retiming is enabled, the delay line is a chain of flip-flops.  xl_area=[1 1 0 0 0 0 0]  block_version=VER_STRING_GOES_HERE
  Inverter : xbsIndex_r4/Inverter  en=off  latency=0  dbl_ovrd=off  block_type=inv
      settings: xl_area=[0 0 0 0 0 0 0]  block_version=VER_STRING_GOES_HERE
  Logical1 : xbsIndex_r4/Logical  logical_function=AND  inputs=2  en=off  latency=0  precision=Full  arith_type=Unsigned  n_bits=8  bin_pt=2  align_bp=on  dbl_ovrd=off  block_type=logical
      settings: xl_area=[1 0 0 1 0 0 0]  block_version=VER_STRING_GOES_HERE
  Q : Outport
  wires:
  Delay/1 -> Inverter/1
  Inverter/1 -> Logical1/1
  Logical1/1 -> Q/1
  D/1 -> Delay/1, Logical1/2

== system w3_warplab_agc/Ctrl/Posedge2 ==
  note: Rising Edge Detection
  D : Inport
  Delay : xbsIndex_r4/Delay  rst=off  infoeditControl=Selection of Reset will increase slice count due to use of real FFs and instead of SRLs  en=off  latency=1  dbl_ovrd=off  reg_retiming=off  block_type=delay
      settings: infoedit=Hardware notes: A delay line is a chain, each link of which is an SRL16 followed by a flip-flop. If register retiming is enabled, the delay line is a chain of flip-flops.  xl_area=[1 1 0 0 0 0 0]  block_version=VER_STRING_GOES_HERE
  Inverter : xbsIndex_r4/Inverter  en=off  latency=0  dbl_ovrd=off  block_type=inv
      settings: xl_area=[0 0 0 0 0 0 0]  block_version=VER_STRING_GOES_HERE
  Logical1 : xbsIndex_r4/Logical  logical_function=AND  inputs=2  en=off  latency=0  precision=Full  arith_type=Unsigned  n_bits=8  bin_pt=2  align_bp=on  dbl_ovrd=off  block_type=logical
      settings: xl_area=[1 0 0 1 0 0 0]  block_version=VER_STRING_GOES_HERE
  Q : Outport
  wires:
  D/1 -> Logical1/2, Delay/1
  Logical1/1 -> Q/1
  Inverter/1 -> Logical1/1
  Delay/1 -> Inverter/1

== system w3_warplab_agc/Ctrl/Posedge3 ==
  note: Rising Edge Detection
  D : Inport
  Delay : xbsIndex_r4/Delay  rst=off  infoeditControl=Selection of Reset will increase slice count due to use of real FFs and instead of SRLs  en=off  latency=1  dbl_ovrd=off  reg_retiming=off  block_type=delay
      settings: infoedit=Hardware notes: A delay line is a chain, each link of which is an SRL16 followed by a flip-flop. If register retiming is enabled, the delay line is a chain of flip-flops.  xl_area=[1 1 0 0 0 0 0]  block_version=VER_STRING_GOES_HERE
  Inverter : xbsIndex_r4/Inverter  en=off  latency=0  dbl_ovrd=off  block_type=inv
      settings: xl_area=[0 0 0 0 0 0 0]  block_version=VER_STRING_GOES_HERE
  Logical1 : xbsIndex_r4/Logical  logical_function=AND  inputs=2  en=off  latency=0  precision=Full  arith_type=Unsigned  n_bits=8  bin_pt=2  align_bp=on  dbl_ovrd=off  block_type=logical
      settings: xl_area=[1 0 0 1 0 0 0]  block_version=VER_STRING_GOES_HERE
  Q : Outport
  wires:
  D/1 -> Logical1/2, Delay/1
  Logical1/1 -> Q/1
  Inverter/1 -> Logical1/1
  Delay/1 -> Inverter/1

== system w3_warplab_agc/Ctrl/Posedge4 ==
  note: Rising Edge Detection
  D : Inport
  Delay : xbsIndex_r4/Delay  rst=off  infoeditControl=Selection of Reset will increase slice count due to use of real FFs and instead of SRLs  en=off  latency=1  dbl_ovrd=off  reg_retiming=off  block_type=delay
      settings: infoedit=Hardware notes: A delay line is a chain, each link of which is an SRL16 followed by a flip-flop. If register retiming is enabled, the delay line is a chain of flip-flops.  xl_area=[1 1 0 0 0 0 0]  block_version=VER_STRING_GOES_HERE
  Inverter : xbsIndex_r4/Inverter  en=off  latency=0  dbl_ovrd=off  block_type=inv
      settings: xl_area=[0 0 0 0 0 0 0]  block_version=VER_STRING_GOES_HERE
  Logical1 : xbsIndex_r4/Logical  logical_function=AND  inputs=2  en=off  latency=0  precision=Full  arith_type=Unsigned  n_bits=8  bin_pt=2  align_bp=on  dbl_ovrd=off  block_type=logical
      settings: xl_area=[1 0 0 1 0 0 0]  block_version=VER_STRING_GOES_HERE
  Q : Outport
  wires:
  Delay/1 -> Inverter/1
  Inverter/1 -> Logical1/1
  Logical1/1 -> Q/1
  D/1 -> Delay/1, Logical1/2

== system w3_warplab_agc/Ctrl/Posedge5 ==
  note: Rising Edge Detection
  D : Inport
  Delay : xbsIndex_r4/Delay  rst=off  infoeditControl=Selection of Reset will increase slice count due to use of real FFs and instead of SRLs  en=off  latency=1  dbl_ovrd=off  reg_retiming=off  block_type=delay
      settings: infoedit=Hardware notes: A delay line is a chain, each link of which is an SRL16 followed by a flip-flop. If register retiming is enabled, the delay line is a chain of flip-flops.  xl_area=[1 1 0 0 0 0 0]  block_version=VER_STRING_GOES_HERE
  Inverter : xbsIndex_r4/Inverter  en=off  latency=0  dbl_ovrd=off  block_type=inv
      settings: xl_area=[0 0 0 0 0 0 0]  block_version=VER_STRING_GOES_HERE
  Logical1 : xbsIndex_r4/Logical  logical_function=AND  inputs=2  en=off  latency=0  precision=Full  arith_type=Unsigned  n_bits=8  bin_pt=2  align_bp=on  dbl_ovrd=off  block_type=logical
      settings: xl_area=[1 0 0 1 0 0 0]  block_version=VER_STRING_GOES_HERE
  Q : Outport
  wires:
  D/1 -> Logical1/2, Delay/1
  Logical1/1 -> Q/1
  Inverter/1 -> Logical1/1
  Delay/1 -> Inverter/1

== system w3_warplab_agc/Ctrl/Posedge6 ==
  note: Rising Edge Detection
  D : Inport
  Delay : xbsIndex_r4/Delay  rst=off  infoeditControl=Selection of Reset will increase slice count due to use of real FFs and instead of SRLs  en=off  latency=1  dbl_ovrd=off  reg_retiming=off  block_type=delay
      settings: infoedit=Hardware notes: A delay line is a chain, each link of which is an SRL16 followed by a flip-flop. If register retiming is enabled, the delay line is a chain of flip-flops.  xl_area=[1 1 0 0 0 0 0]  block_version=VER_STRING_GOES_HERE
  Inverter : xbsIndex_r4/Inverter  en=off  latency=0  dbl_ovrd=off  block_type=inv
      settings: xl_area=[0 0 0 0 0 0 0]  block_version=VER_STRING_GOES_HERE
  Logical1 : xbsIndex_r4/Logical  logical_function=AND  inputs=2  en=off  latency=0  precision=Full  arith_type=Unsigned  n_bits=8  bin_pt=2  align_bp=on  dbl_ovrd=off  block_type=logical
      settings: xl_area=[1 0 0 1 0 0 0]  block_version=VER_STRING_GOES_HERE
  Q : Outport
  wires:
  D/1 -> Logical1/2, Delay/1
  Logical1/1 -> Q/1
  Inverter/1 -> Logical1/1
  Delay/1 -> Inverter/1

== system w3_warplab_agc/Ctrl/Posedge7 ==
  note: Rising Edge Detection
  D : Inport
  Delay : xbsIndex_r4/Delay  rst=off  infoeditControl=Selection of Reset will increase slice count due to use of real FFs and instead of SRLs  en=off  latency=1  dbl_ovrd=off  reg_retiming=off  block_type=delay
      settings: infoedit=Hardware notes: A delay line is a chain, each link of which is an SRL16 followed by a flip-flop. If register retiming is enabled, the delay line is a chain of flip-flops.  xl_area=[1 1 0 0 0 0 0]  block_version=VER_STRING_GOES_HERE
  Inverter : xbsIndex_r4/Inverter  en=off  latency=0  dbl_ovrd=off  block_type=inv
      settings: xl_area=[0 0 0 0 0 0 0]  block_version=VER_STRING_GOES_HERE
  Logical1 : xbsIndex_r4/Logical  logical_function=AND  inputs=2  en=off  latency=0  precision=Full  arith_type=Unsigned  n_bits=8  bin_pt=2  align_bp=on  dbl_ovrd=off  block_type=logical
      settings: xl_area=[1 0 0 1 0 0 0]  block_version=VER_STRING_GOES_HERE
  Q : Outport
  wires:
  D/1 -> Logical1/2, Delay/1
  Logical1/1 -> Q/1
  Inverter/1 -> Logical1/1
  Delay/1 -> Inverter/1

== system w3_warplab_agc/Ctrl/Posedge8 ==
  note: Rising Edge Detection
  D : Inport
  Delay : xbsIndex_r4/Delay  rst=off  infoeditControl=Selection of Reset will increase slice count due to use of real FFs and instead of SRLs  en=off  latency=1  dbl_ovrd=off  reg_retiming=off  block_type=delay
      settings: infoedit=Hardware notes: A delay line is a chain, each link of which is an SRL16 followed by a flip-flop. If register retiming is enabled, the delay line is a chain of flip-flops.  xl_area=[1 1 0 0 0 0 0]  block_version=VER_STRING_GOES_HERE
  Inverter : xbsIndex_r4/Inverter  en=off  latency=0  dbl_ovrd=off  block_type=inv
      settings: xl_area=[0 0 0 0 0 0 0]  block_version=VER_STRING_GOES_HERE
  Logical1 : xbsIndex_r4/Logical  logical_function=AND  inputs=2  en=off  latency=0  precision=Full  arith_type=Unsigned  n_bits=8  bin_pt=2  align_bp=on  dbl_ovrd=off  block_type=logical
      settings: xl_area=[1 0 0 1 0 0 0]  block_version=VER_STRING_GOES_HERE
  Q : Outport
  wires:
  Delay/1 -> Inverter/1
  Inverter/1 -> Logical1/1
  Logical1/1 -> Q/1
  D/1 -> Delay/1, Logical1/2

== system w3_warplab_agc/Ctrl/Posedge9 ==
  note: Rising Edge Detection
  D : Inport
  Delay : xbsIndex_r4/Delay  rst=off  infoeditControl=Selection of Reset will increase slice count due to use of real FFs and instead of SRLs  en=off  latency=1  dbl_ovrd=off  reg_retiming=off  block_type=delay
      settings: infoedit=Hardware notes: A delay line is a chain, each link of which is an SRL16 followed by a flip-flop. If register retiming is enabled, the delay line is a chain of flip-flops.  xl_area=[1 1 0 0 0 0 0]  block_version=VER_STRING_GOES_HERE
  Inverter : xbsIndex_r4/Inverter  en=off  latency=0  dbl_ovrd=off  block_type=inv
      settings: xl_area=[0 0 0 0 0 0 0]  block_version=VER_STRING_GOES_HERE
  Logical1 : xbsIndex_r4/Logical  logical_function=AND  inputs=2  en=off  latency=0  precision=Full  arith_type=Unsigned  n_bits=8  bin_pt=2  align_bp=on  dbl_ovrd=off  block_type=logical
      settings: xl_area=[1 0 0 1 0 0 0]  block_version=VER_STRING_GOES_HERE
  Q : Outport
  wires:
  Delay/1 -> Inverter/1
  Inverter/1 -> Logical1/1
  Logical1/1 -> Q/1
  D/1 -> Delay/1, Logical1/2
